simulink model "stable_sim"  (R2021a)
settings: Solver=FixedStepAuto  StartTime=0.0  StopTime=20  FixedStep=0.002  RelTol=1e-3
values from neighbouring files (symbols this model uses):
  alpha_0 = 0    [optimised.mat]    (also in stable_simulator.m)
  bp = -0.000688404850643    [optimised.mat]    (also in qube2_rotpen_param.m = 5e-05; qube2_rotpen_param_adjusted.m = -0.00087613)
  br = 0.00579712620159    [optimised.mat]    (also in qube2_rotpen_param.m = 0.001; qube2_rotpen_param_adjusted.m = 0.0066047)
  g = 9.81    [optimised.mat]    (also in qube2_rotpen_param.m; qube2_rotpen_param_adjusted.m)
  Jp = 0.000301833422623    [optimised.mat]    (also in qube2_rotpen_param.m = 0.000133128; qube2_rotpen_param_adjusted.m = 0.0004295)
  Jr = 0.0017561686084    [optimised.mat]    (also in qube2_rotpen_param.m = 0.000228791666667; qube2_rotpen_param_adjusted.m = 0.0024586)
  l = 0.0461368890877    [optimised.mat]    (also in qube2_rotpen_param.m = 0.0645; qube2_rotpen_param_adjusted.m = 0.044321)
  mp = 0.038227720685    [optimised.mat]    (also in qube2_rotpen_param.m = 0.024; qube2_rotpen_param_adjusted.m = 0.045211)
  r = 0.372401705528    [optimised.mat]    (also in qube2_rotpen_param.m = 0.085; qube2_rotpen_param_adjusted.m = 0.47498)
  thetadd_max = 72.7865151285    [optimised.mat]    (also in qube2_rotpen_param.m = 72.8464760517; qube2_rotpen_param_adjusted.m = 72.8465)
settings Model: OrderedModelArguments=off  Creator=willi

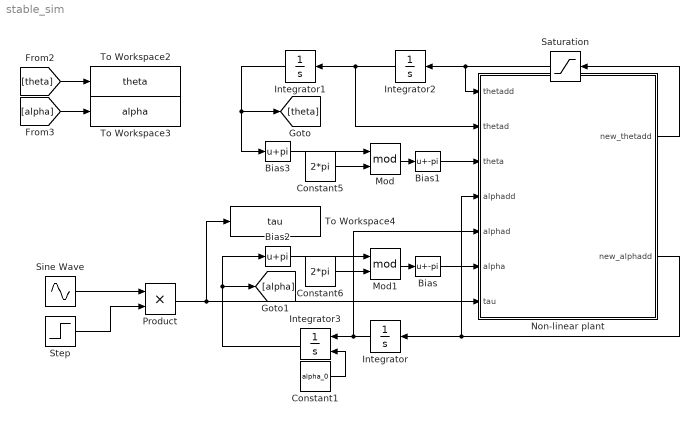
== system stable_sim ==
  Bias : Bias  Bias=-pi
  Bias1 : Bias  Bias=-pi
  Bias2 : Bias  Bias=pi
  Bias3 : Bias  Bias=pi
  Constant1 : Constant  Value=alpha_0
  Constant5 : Constant  Value=2*pi
  Constant6 : Constant  Value=2*pi
  Integrator : Integrator
  Integrator1 : Integrator
  Integrator2 : Integrator
  Integrator3 : Integrator  InitialConditionSource=external
  Mod : Math  Operator=mod  SaturateOnIntegerOverflow=on
  Mod1 : Math  Operator=mod  SaturateOnIntegerOverflow=on
  Non-linear plant : Subsystem
  Product : Product
  Saturation : Saturate  UpperLimit=thetadd_max  LowerLimit=-thetadd_max
  Sine Wave : Sin  Amplitude=0.005  Frequency=20  SampleTime=0
  Step : Step  Time=10  Before=1  After=0  SampleTime=0
  To Workspace2 : ToWorkspace  VariableName=theta  SaveFormat=Timeseries  SampleTime=-1
  To Workspace3 : ToWorkspace  VariableName=alpha  SaveFormat=Timeseries  SampleTime=-1
  To Workspace4 : ToWorkspace  VariableName=tau  SaveFormat=Timeseries  SampleTime=-1
  wires:
  Non-linear plant/1(new_thetadd) -> Saturation/1
  Non-linear plant/2(new_alphadd) -> Non-linear plant/4(alphadd), Integrator/1
  Constant1/1 -> Integrator3/2
  Constant5/1 -> Mod/2
  Mod/1 -> Bias1/1
  Integrator1/1 -> [theta], Bias3/1
  Mod1/1 -> Bias/1
  Constant6/1 -> Mod1/2
  Integrator3/1 -> [alpha], Bias2/1
  Bias3/1 -> Mod/1
  Bias2/1 -> Mod1/1
  Bias1/1 -> Non-linear plant/3(theta)
  Integrator/1 -> Non-linear plant/5(alphad), Integrator3/1
  Bias/1 -> Non-linear plant/6(alpha)
  Integrator2/1 -> Non-linear plant/2(thetad), Integrator1/1
  Saturation/1 -> Non-linear plant/1(thetadd), Integrator2/1
  [theta] -> To Workspace2/1
  [alpha] -> To Workspace3/1
  Product/1 -> To Workspace4/1, Non-linear plant/7(tau)
  Sine Wave/1 -> Product/1
  Step/1 -> Product/2

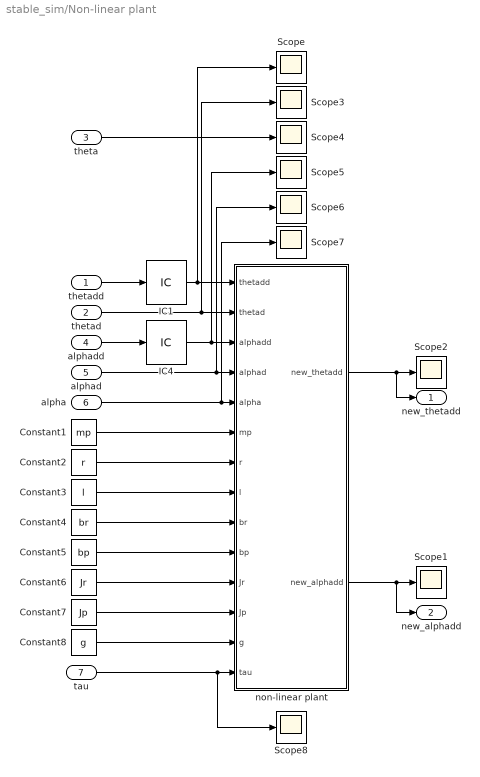
== system stable_sim/Non-linear plant ==
  thetadd : Inport
  thetad : Inport  Port=2
  theta : Inport  Port=3
  alphadd : Inport  Port=4
  alphad : Inport  Port=5
  alpha : Inport  Port=6
  tau : Inport  Port=7
  Constant1 : Constant  Value=mp
  Constant2 : Constant  Value=r
  Constant3 : Constant  Value=l
  Constant4 : Constant  Value=br
  Constant5 : Constant  Value=bp
  Constant6 : Constant  Value=Jr
  Constant7 : Constant  Value=Jp
  Constant8 : Constant  Value=g
  IC1 : InitialCondition  Value=0
  IC4 : InitialCondition  Value=0
  Scope{,1..8} (9 alike) : Scope
  non-linear plant : MATLAB Function  TreatAsAtomicUnit=on
  new_thetadd : Outport
  new_alphadd : Outport  Port=2
  wires:
  Constant3/1 -> non-linear plant/8(l)
  Constant2/1 -> non-linear plant/7(r)
  alphad/1 -> Scope6/1, non-linear plant/4(alphad)
  non-linear plant/1(new_thetadd) -> new_thetadd/1, Scope2/1
  alpha/1 -> Scope7/1, non-linear plant/5(alpha)
  Constant1/1 -> non-linear plant/6(mp)
  thetad/1 -> Scope3/1, non-linear plant/2(thetad)
  Constant7/1 -> non-linear plant/12(Jp)
  non-linear plant/2(new_alphadd) -> new_alphadd/1, Scope1/1
  Constant5/1 -> non-linear plant/10(bp)
  theta/1 -> Scope4/1
  Constant4/1 -> non-linear plant/9(br)
  Constant8/1 -> non-linear plant/13(g)
  Constant6/1 -> non-linear plant/11(Jr)
  thetadd/1 -> IC1/1
  alphadd/1 -> IC4/1
  IC1/1 -> Scope/1, non-linear plant/1(thetadd)
  IC4/1 -> Scope5/1, non-linear plant/3(alphadd)
  tau/1 -> Scope8/1, non-linear plant/14(tau)

== matlab function stable_sim/Non-linear plant/non-linear plant ==
  data: thetadd input; thetad input; new_thetadd output; alphadd input; alphad input; alpha input; mp input; r input; l input; br input; bp input; Jr input; Jp input; g input; tau input; new_alphadd output
function [new_thetadd, new_alphadd]= fcn(thetadd, thetad, alphadd, alphad, alpha, mp, r, l, br, bp, Jr, Jp, g, tau)

new_alphadd = (-bp*alphad - mp*g*l*sin(alpha) + Jp*(thetad^2)*sin(alpha)*cos(alpha) - mp*l*r*thetadd*cos(alpha)) / Jp;
new_thetadd = (tau - br*thetad + mp*l*r*(alphad^2)*sin(alpha) - 2*Jp*alphad*thetad*sin(alpha)*cos(alpha) - mp*l*r*alphadd*cos(alpha)) / (Jr+Jp*(sin(alpha)^2));
